simulink model "test_Rehamove3_NetworkInterface"  (R2016b)
settings: Solver=FixedStepDiscrete  StartTime=0.0  StopTime=inf  FixedStep=0.05  RelTol=1e-3
libraries: LIB_NetwokInterface x1, Lib_RehaMove3 x1
settings Model: SimulationMode=external  ExtModeTrigDuration=10000  Creator=constantin  LastModifiedBy=valtin
settings DataIOCC: LimitDataPoints=on  SaveFormat=Array
settings OptimizationCC: ExpressionDepthLimit=2147483647  LifeSpan=1
settings DebuggingCC: UnderspecifiedInitializationDetection=Classic  MergeDetectMultiDrivingBlocksExec=none  SolverPrmCheckMsg=warning  StateNameClashWarn=warning  SFUnexpectedBacktrackingDiag=warning  SFNoUnconditionalDefaultTransitionDiag=warning  SFExecutionAtInitializationDiag=none
settings HardwareCC: ProdBitPerPointer=32  ProdBitPerSizeT=32  ProdBitPerPtrDiffT=32  ProdLargestAtomicFloat=None  ProdIntDivRoundTo=Undefined  ProdEndianess=Unspecified  ProdWordSize=32  ProdHWDeviceType=32-bit Generic
settings ModelReferenceCC: PropagateSignalLabelsOutOfModel=off
settings SFSimCC: SimParseCustomCode=off
settings RTWCC: SystemTargetFile=ert_linux.tlc  MakeCommand=make_rtw OPTS=-DWITH_HW OPTIMIZATION_FLAGS=-O3  TemplateMakefile=ert_linux.tmf  Description=Linux Embedded Coder  TargetLang=C++
settings CodeAppCC: IgnoreCustomStorageClasses=off  CustomSymbolStrType=$N$R$M  InternalIdentifier=Classic
settings STFCustomTargetCC: ModelReferenceCompliant=off  GeneratePreprocessorConditionals=Disable all  CombineOutputUpdateFcns=on  ERTCustomFileBanners=on  SupportComplex=off  RemoveResetFunc=on  SupportVariableSizeSignals=on  MATLABClassNameForMDSCustomization=Simulink.SoftwareTarget.ERTCustomization  GRTInterface=off  SystemTargetFile=ert_linux.tlc
settings ERTTargetCC: ModelReferenceCompliant=off  ParMdlRefBuildCompliant=off  CompOptLevelCompliant=off  ConcurrentExecutionCompliant=off  GeneratePreprocessorConditionals=Disable all  ERTFirstTimeCompliant=off  SupportComplex=off  SupportContinuousTime=on  SupportNonInlinedSFcns=on  SupportVariableSizeSignals=on  ModelStepFunctionPrototypeControlCompliant=off  CPPClassGenCompliant=off  UseToolchainInfoCompliant=off  ExtMode=on  MultiInstanceErrorCode=None  ERTCustomFileTemplate=ert_linux_file_process.tlc  ConvertIfToSwitch=off  SuppressUnreachableDefaultCases=off
settings ConfigComp: CovMetricSettings=dw  CovHtmlReporting=on  CovSaveCumulativeToWorkspaceVar=on  CovSaveSingleToWorkspaceVar=on  CovExternalEMLEnable=off  CovSFcnEnable=off
settings ConfigurationSet: Description=SimMechanics 2G

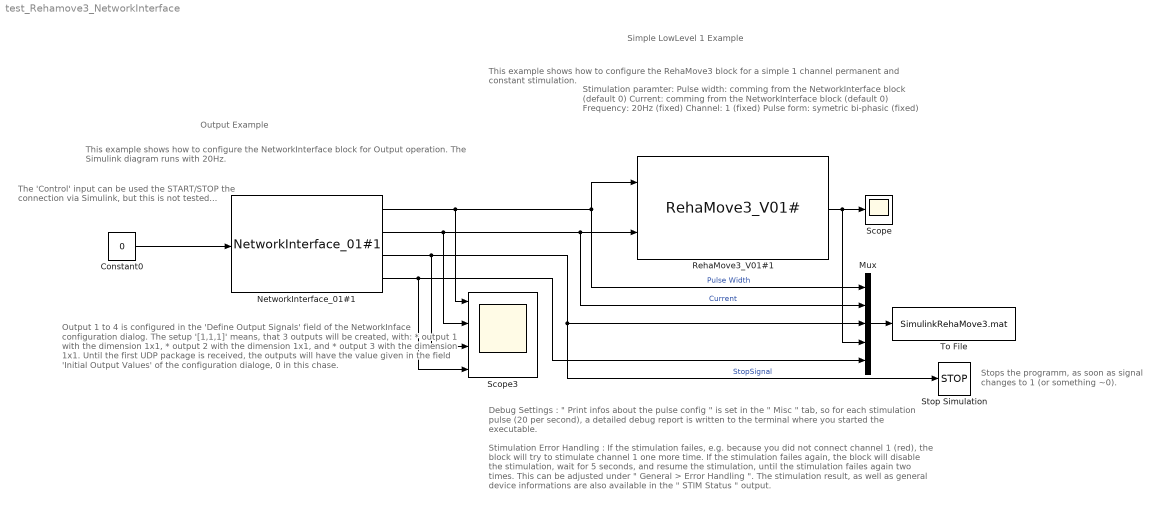
== system test_Rehamove3_NetworkInterface ==
  note: Output Example
  note: This example shows how to configure the NetworkInterface block for Output operation.
      | The Simulink diagram runs with 20Hz.
  note: The 'Control' input can be used the START/STOP
      | the connection via Simulink, but this is not tested...
  note: Output 1 to 4 is configured in the 'Define Output Signals' field of the NetworkInface
      | configuration dialog. The setup '[1,1,1]' means, that 3 outputs will be created, with:
      |  * output 1 with the dimension 1x1,
      |  * output 2 with the dimension 1x1, and
      |  * output 3 with the dimension 1x1.
      |
      | Until the first UDP package is received, the outputs will have the value given in the field
      | 'Initial Output Values' of the configuration dialoge, 0 in this chase.
  note: Stops the programm, as soon as signal
      | changes to 1 (or something ~0).
  note: Stimulation Error Handling :
      | If the stimulation failes, e.g. because you did not connect channel 1 (red), the block will try to stimulate channel 1 one more time.
      | If the stimulation failes again, the block will disable the stimulation, wait for 5 seconds, and resume the stimulation,
      | until the stimulation failes again two times. This can be adjusted under " General > Error Handling ".
      | The stimulation result, as well as general device informations are also available in the " STIM Status " output.
  note: Debug Settings : " Print infos about the pulse config " is set in the " Misc " tab, so for each stimulation pulse (20 per second),
      | a detailed debug report is written to the terminal where you started the executable.
  note: Stimulation paramter:
      | Pulse width: comming from the NetworkInterface block (default 0)
      | Current: comming from the NetworkInterface block (default 0)
      | Frequency: 20Hz (fixed)
      | Channel: 1 (fixed)
      | Pulse form: symetric bi-phasic (fixed)
  note: This example shows how to configure the RehaMove3 block for a simple 1 channel permanent and constant stimulation.
  note: Simple LowLevel 1 Example
  Constant0 : Constant  Value=0  OutDataTypeStr=double  SampleTime=-1
  Mux : Mux  Inputs=5
  NetworkInterface_01#1 : LIB_NetwokInterface/NetworkInterface_01#1  inputs=0  outputs=[1,1,1]  initialOutputValues=0  SampleTime=-1  useUDP=on  startConnection=on  localPort=20000  remoteIP='127.0.0.1'  remotePort=20001
  RehaMove3_V01#1 : Lib_RehaMove3/RehaMove3_V01#  stimDevicePath=/dev/ttyUSB0  stimChannels=[ 1 ]  stimFrequency=20  stimRehaMoveProProtocol="Use the LowLevel protocol   -> Each stimulation pulse is send separatly."  stimMaxCurrent=90  stimMaxPulsWidth=500  stimBlockID=STIM1  stimTextSampleTime=0.05s (based on stimulation frequency)  SampleTime=0.05  stimThreadInit=on  stimThreadData=on  stimAbortError=2  stimTestAgain=5  llPulseShape=[0]  llNumberOfParts=1  llMaxStimVoltage=90V  llActivateDenervation=off  mlFStim=20  mlFStimDynamic=on  mlFKeepAlive=0.76923  mlUseSoftStart=on  mlUseRamps=off  mlRampsUpdates=3  mlRampsZeroUpdates=0  miscPrintBlockParam=off  miscPrintDeviceInfos=off  miscPrintSendInfos=off  miscPrintReceiveInfos=off  miscPrintInitInfos=off  miscPrintStimInfos=on  miscPrintRMPInitSettings=on  miscPrintCorrectionChargeWarnings=on  miscPrintSequenceErrors=on  miscPrintTimingErrors=on  miscUseColors=on  miscPrintStats=on  miscEnableAdvancedSettings=off  miscDisableVersionCheck=off
  Scope : Scope
  Scope3 : Scope  NumInputPorts=4
  Stop Simulation : Stop
  To File : ToFile  Filename=SimulinkRehaMove3.mat  MatrixName=rmConfig
  wires:
  Constant0/1 -> NetworkInterface_01#1/1
  NetworkInterface_01#1/4 -> Mux/5, Scope3/4
  Mux/1 -> To File/1
  RehaMove3_V01#1/1 -> Mux/4, Scope/1
  NetworkInterface_01#1/2 -> Scope3/2, Mux/2, RehaMove3_V01#1/2  "Current"
  NetworkInterface_01#1/1 -> Scope3/1, RehaMove3_V01#1/1, Mux/1  "Pulse Width"
  NetworkInterface_01#1/3 -> Scope3/3, Mux/3, Stop Simulation/1  "StopSignal"
